simulink model "M_DYN_Thrust"  (R2022a)
settings: Solver=ode4  StartTime=0.0  StopTime=0.04  FixedStep=0.01  RelTol=1e-3
undefined symbols (not defined in the file or in its folder): DiscIntNeverNeededParam
libraries: aerolibatmos2 x1, aerolibasang x1
settings Model: Creator=ASCL  LastModifiedBy=ASCL
settings DataIOCC: SaveOutput=off  SignalLogging=off  DSMLogging=off  SaveTime=off  ReturnWorkspaceOutputs=off
settings OptimizationCC: BlockReduction=off  DefaultParameterBehavior=Inlined  UseDivisionForNetSlopeComputation=on  GainParamInheritBuiltInType=on  UseFloatMulNetSlope=on  ExpressionFolding=off  PassReuseOutputArgsAs=Individual arguments  ZeroExternalMemoryAtStartup=off  ZeroInternalMemoryAtStartup=off  EfficientFloat2IntCast=on  LifeSpan=inf  OptimizeBlockOrder=speed  DifferentSizesBufferReuse=on  EfficientTunableParamExpr=on
settings DebuggingCC: SignalInfNanChecking=warning  ReadBeforeWriteMsg=EnableAllAsError  WriteAfterWriteMsg=EnableAllAsError  WriteAfterReadMsg=EnableAllAsError  IntegerOverflowMsg=error  ParameterTunabilityLossMsg=error  UniqueDataStoreMsg=error  AssertControl=DisableAll  NonBusSignalsTreatedAsBus=error  SFInvalidInputDataAccessInChartInitDiag=error  SFTransitionOutsideNaturalParentDiag=error  SFUnreachableExecutionPathDiag=error  SFUndirectedBroadcastEventsDiag=error  IntegerSaturationMsg=error
settings HardwareCC: ProdBitPerPointer=32  ProdBitPerSizeT=32  ProdBitPerPtrDiffT=32  ProdLargestAtomicInteger=Long  ProdLargestAtomicFloat=Double  ProdEndianess=BigEndian  ProdWordSize=32  ProdLongLongMode=on  ProdHWDeviceType=Freescale->MPC83xx
settings ModelReferenceCC: ModelReferenceNumInstancesAllowed=Single
settings SFSimCC: CompileTimeRecursionLimit=0  EnableRuntimeRecursion=off  MATLABDynamicMemAlloc=off
settings RTWCC: SystemTargetFile=ert.tlc  TemplateMakefile=ert_default_tmf  GenerateReport=on  BuildConfiguration=Faster Runs  IncludeHyperlinkInReport=on  LaunchReport=on  GenerateTraceInfo=on  GenerateTraceReport=on  GenerateTraceReportSl=on  GenerateTraceReportSf=on  GenerateTraceReportEml=on
settings CodeAppCC: ForceParamTrailComments=on  IgnoreCustomStorageClasses=off  OperatorAnnotations=on  SimulinkDataObjDesc=on  SFDataObjDesc=on  MATLABFcnDesc=on  InsertBlockDesc=on  StateflowObjectComments=on  MATLABSourceComments=on  EnableCustomComments=on  InlinedPrmAccess=Macros  ReqsInCode=on
settings ERTTargetCC: TargetLangStandard=C99 (ISO)  UtilityFuncGeneration=Shared location  GenerateSampleERTMain=on  IncludeMdlTerminateFcn=off  CombineSignalStateStructs=on  SupportNonFinite=off  SupportVariableSizeSignals=on  ParenthesesLevel=Standards  CastingMode=Standards  GenerateSharedConstants=off  InlinedParameterPlacement=NonHierarchical  ERTCustomFileTemplate=example_file_process.tlc  RateTransitionBlockCode=Function  PreserveIfCondition=on  ConvertIfToSwitch=off  EnableSignedLeftShifts=off  EnableSignedRightShifts=off

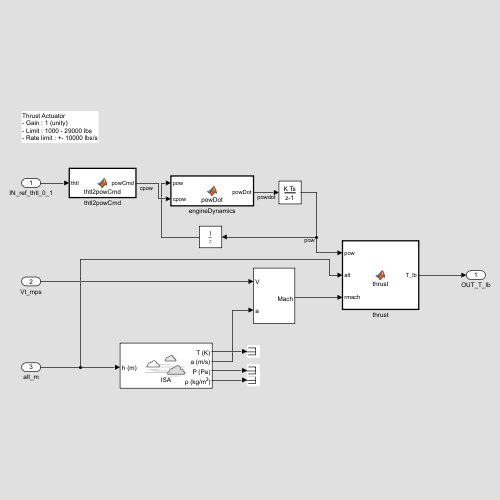
[thumbnail: Simulink's stored preview of the top-level diagram]
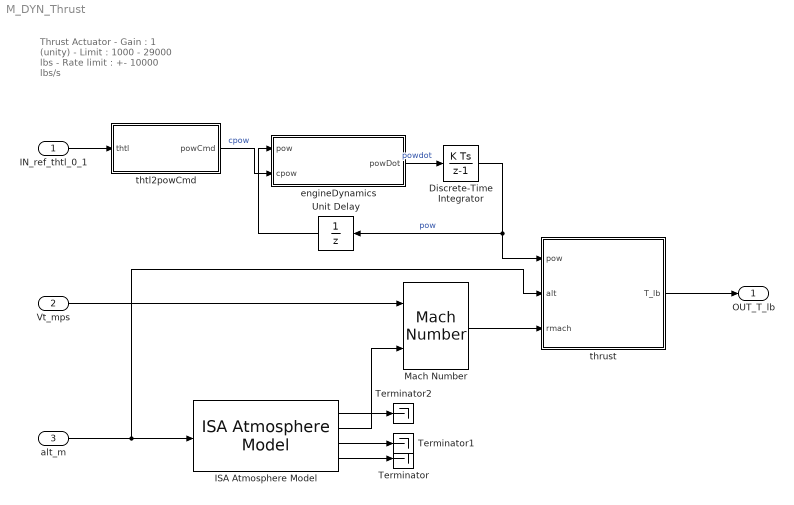
== system M_DYN_Thrust ==
  note: Thrust Actuator
      | - Gain : 1 (unity)
      | - Limit : 1000 - 29000 lbs
      | - Rate limit : +- 10000 lbs/s
  IN_ref_thtl_0_1 : Inport  OutMin=0  OutMax=1  OutDataTypeStr=double  Interpolate=off
  Vt_mps : Inport  Port=2  Interpolate=off
  alt_m : Inport  Port=3  Interpolate=off
  Discrete-Time Integrator : DiscreteIntegrator  SampleTime=0.01  ICPrevOutput=DiscIntNeverNeededParam  ICPrevScaledInput=DiscIntNeverNeededParam
  ISA Atmosphere Model : aerolibatmos2/ISA Atmosphere Model  custom=off  g=9.80665  gamma=1.4  R=287.0531  L=0.0065  h_trop=11000  h_strat=20000  rho0=1.225  P0=101325  T0=288.15  h0=0
  Mach Number : aerolibasang/Mach Number
      settings: SourceProductBaseCode=AE
  Terminator : Terminator
  Terminator1 : Terminator
  Terminator2 : Terminator
  Unit Delay : UnitDelay  SampleTime=-1  HasFrameUpgradeWarning=on
  engineDynamics : MATLAB Function  TreatAsAtomicUnit=on
  thrust : MATLAB Function  TreatAsAtomicUnit=on
  thtl2powCmd : MATLAB Function  TreatAsAtomicUnit=on
  OUT_T_lb : Outport  OutDataTypeStr=double  VectorParamsAs1DForOutWhenUnconnected=off
  wires:
  thrust/1(T_lb) -> OUT_T_lb/1
  IN_ref_thtl_0_1/1 -> thtl2powCmd/1(thtl)
  Unit Delay/1 -> engineDynamics/1(pow)
  engineDynamics/1(powDot) -> Discrete-Time Integrator/1  "powdot"
  Discrete-Time Integrator/1 -> thrust/1(pow), Unit Delay/1  "pow"
  alt_m/1 -> ISA Atmosphere Model/1, thrust/2(alt)
  Vt_mps/1 -> Mach Number/1
  Mach Number/1 -> thrust/3(rmach)
  ISA Atmosphere Model/2 -> Mach Number/2
  ISA Atmosphere Model/1 -> Terminator2/1
  ISA Atmosphere Model/3 -> Terminator1/1
  ISA Atmosphere Model/4 -> Terminator/1
  thtl2powCmd/1(powCmd) -> engineDynamics/2(cpow)  "cpow"

== matlab function M_DYN_Thrust/engineDynamics ==
  data: pow input; cpow input; powDot output
function powDot = powDot(pow, cpow)
if (cpow>=0.5)
    if (pow>=0.5)
        t = 5;
        p2 = cpow;
    else
        p2 = 0.6;
        t = tc(p2-pow);
    end
else
    if (pow>=0.5)
        t = 5;
        p2 = 0.4;
    else
        p2 = cpow;
        t = tc(p2-pow);
    end
end
powDot = t * (p2-pow);

end

function tau_aux = tc(pow_diff)

if (pow_diff <= 0.25)
    tau_aux = 1.0;
elseif (pow_diff >= 0.5)
    tau_aux = 0.1;
else
    tau_aux = 1.9 - 3.6 * pow_diff;
end

end

== matlab function M_DYN_Thrust/thtl2powCmd ==
  data: thtl input; powCmd output
function powCmd = thtl2powCmd(thtl)
% thtl2powCmd
% --- Input ---
% thtl: [0-1]
% --- Output ---
% powCmd: [0-1]

if ( thtl <= 0.77 )
    powCmd = 0.6494 * thtl;
else
    powCmd = 2.1738 * thtl - 1.1738;
end

== matlab function M_DYN_Thrust/thrust ==
  data: pow input; T_lb output; alt input; rmach input
function T_lb=thrust(pow,alt,rmach)

% adding a check for neg velocity
if rmach<0
    rmach=0;
end

a=[1060 670 880 1140 1500 1860
    635 425 690 1010 1330 1700
    60 25 345 755 1130 1525
    -1020 -170 -300 350 910 1360
    -2700 -1900 -1300 -247 600 1100
    -3600 -1400 -595 -342 -200 700]';

b=[12680 9150 6200 3950 2450 1400
    12680 9150 6313 4040 2470 1400
    12610 9312 6610 4290 2600 1560
    12640 9839 7090 4660 2840 1660
    12390 10176 7750 5320 3250 1930
    11680 9848 8050 6100 3800 2310]';

c=[20000 15000 10800 7000 4000 2500
    21420 15700 11225 7323 4435 2600
    22700 16860 12250 8154 5000 2835
    24240 18910 13760 9285 5700 3215
    26070 21075 15975 11115 6860 3950
    28886 23319 18300 13484 8642 5057]';

if(alt<0),alt=0.01;end
h=.0001*(alt*3.28084);
i=fix(h);
if(i>=5),i=4;end
dh=h-i;
rm=5*rmach;
m=fix(rm);
if(m>=5);m=4;end

dm = rm - m;
cdh = 1 - dh;

i=i+1;
m=m+1;

s=b(i,m)*cdh+b(i+1,m)*dh;
t=b(i,m+1)*cdh+b(i+1,m+1)*dh;
tmil=s+(t-s)*dm;

if(pow<0.5)
    s=a(i,m)*cdh+a(i+1,m)*dh;
    t=a(i,m+1)*cdh+a(i+1,m+1)*dh;
    tidl=s+(t-s)*dm;
    T_lb=tidl+(tmil-tidl)*pow*2;
else
    s=c(i,m)*cdh+c(i+1,m)*dh;
    t=c(i,m+1)*cdh+c(i+1,m+1)*dh;
    tmax=s+(t-s)*dm;
    T_lb=tmil+(tmax-tmil)*(pow-0.5)*2;
end
